simulink model "Remedy_WWTP"  (R2022a)
settings: Solver=ode23t  StartTime=0.0  StopTime=inf  FixedStep=1E-4  MaxStep=100  RelTol=1e-4  EnableMultiTasking=on
InitFcn:
  | iniASU_UNIT
undefined symbols (not defined in the file or in its folder): Arrhenius, Cineticos20, Esteq, Inf_Const, Param_ASU_D, Param_ASU_N, Param_Settler_Fns, ParamsEsteq, VarManip_D, VarManip_N, VarManip_QRF, x0_D, x0_N
libraries: modbusMatLib x3
settings Model: Creator=iirizar
settings SolverCC: InitialStep=1E-22  MaxConsecutiveMinStep=auto  AlgebraicLoopSolver=TrustRegion  SolverResetMethod=Robust
settings DataIOCC: LimitDataPoints=on  MaxDataPoints=1  SaveFinalState=on  SaveFormat=Array  SignalLoggingSaveFormat=ModelDataLogs  SaveOutput=off  SaveState=on  SignalLogging=off  SaveTime=off  ReturnWorkspaceOutputs=off
settings OptimizationCC: ExpressionDepthLimit=2147483647  LifeSpan=inf
settings DebuggingCC: UnderspecifiedInitializationDetection=Classic  MergeDetectMultiDrivingBlocksExec=none  SolverPrmCheckMsg=warning  FcnCallInpInsideContextMsg=warning  UnconnectedInputMsg=warning  UnconnectedOutputMsg=warning  UnconnectedLineMsg=warning  StateNameClashWarn=warning  SFUnexpectedBacktrackingDiag=warning  SFNoUnconditionalDefaultTransitionDiag=warning  SFExecutionAtInitializationDiag=none  SFMachineParentedDataDiag=warning  ArithmeticOperatorsInVariantConditions=warning
settings HardwareCC: ProdBitPerPointer=32  ProdBitPerSizeT=32  ProdBitPerPtrDiffT=32  ProdLargestAtomicFloat=None  ProdIntDivRoundTo=Undefined  ProdEndianess=Unspecified  ProdWordSize=32  ProdHWDeviceType=32-bit Generic
settings ModelReferenceCC: PropagateSignalLabelsOutOfModel=off
settings SFSimCC: SimUseLocalCustomCode=off  CustomCodeUndefinedFunction=UseInterfaceOnly
settings RTWCC: RTWUseLocalCustomCode=off  DLArmComputeVersion=19.05
settings CodeAppCC: StateflowObjectComments=on
settings GRTTargetCC: TargetLangStandard=C89/C90 (ANSI)  CombineOutputUpdateFcns=off  GRTInterface=on
settings ConfigComp: CovMetricSettings=dw  CovSaveCumulativeToWorkspaceVar=on  CovSaveSingleToWorkspaceVar=on  CovExternalEMLEnable=off

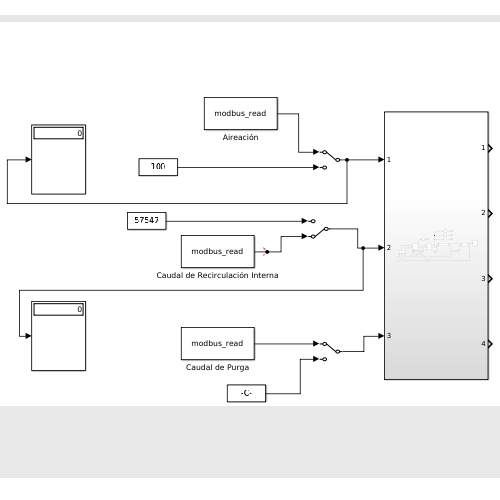
[thumbnail: Simulink's stored preview of the top-level diagram]
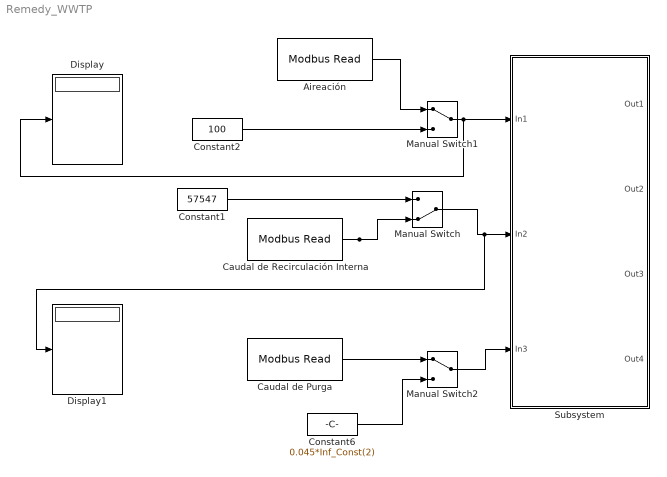
== system Remedy_WWTP ==
  Aireación : modbusMatLib/Modbus Read  registry=2065  ipAddress='openplc'  port=502
  Caudal de Purga : modbusMatLib/Modbus Read  registry=2069  ipAddress='openplc'  port=502
  Caudal de Recirculación Interna : modbusMatLib/Modbus Read  registry=2073  ipAddress='openplc'  port=502
  Constant1 : Constant  Value=57547
  Constant2 : Constant  Value=100
  Constant6 : Constant  Value=0.045*Inf_Const(2)
  Display : Display
  Display1 : Display
  Manual Switch : ManualSwitch  CurrentSetting=0
  Manual Switch1 : ManualSwitch
  Manual Switch2 : ManualSwitch
  Subsystem : Subsystem
  wires:
  Caudal de Recirculación Interna/1 -> Manual Switch/2
  Manual Switch/1 -> Display1/1, Subsystem/2(In2)
  Manual Switch1/1 -> Display/1, Subsystem/1(In1)
  Aireación/1 -> Manual Switch1/1
  Constant2/1 -> Manual Switch1/2
  Constant1/1 -> Manual Switch/1
  Caudal de Purga/1 -> Manual Switch2/1
  Constant6/1 -> Manual Switch2/2
  Manual Switch2/1 -> Subsystem/3(In3)

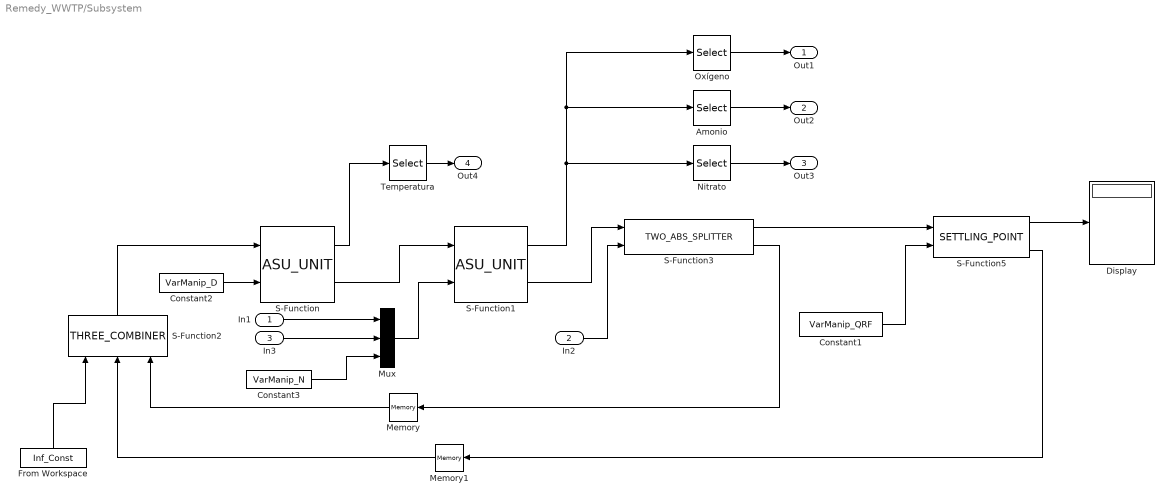
== system Remedy_WWTP/Subsystem ==
  In1 : Inport
  In2 : Inport  Port=2
  In3 : Inport  Port=3
  Amonio : Selector  InputPortWidth=9  IndexOptions=Index vector (dialog)  Indices=[4]  OutputSizes=1
  Constant1 : Constant  Value=VarManip_QRF
  Constant2 : Constant  Value=VarManip_D
  Constant3 : Constant  Value=VarManip_N
  Display : Display
  From Workspace : FromWorkspace  VariableName=Inf_Const  Interpolate=off  OutputAfterFinalValue=Holding final value
  Memory : Memory  InheritSampleTime=on
  Memory1 : Memory  InheritSampleTime=on
  Mux : Mux  Inputs=3
  Nitrato : Selector  InputPortWidth=9  IndexOptions=Index vector (dialog)  Indices=[3]  OutputSizes=1
  Oxígeno : Selector  InputPortWidth=9  IndexOptions=Index vector (dialog)  Indices=[5]  OutputSizes=1
  S-Function : S-Function  FunctionName=ASU_UNIT  Parameters=ParamsEsteq,Cineticos20,Arrhenius,Esteq,Param_ASU_D,x0_D  SFunctionDeploymentMode=off  EnableBusSupport=off
  S-Function1 : S-Function  FunctionName=ASU_UNIT  Parameters=ParamsEsteq,Cineticos20,Arrhenius,Esteq,Param_ASU_N,x0_N  SFunctionDeploymentMode=off  EnableBusSupport=off
  S-Function2 : S-Function  FunctionName=THREE_COMBINER  SFunctionDeploymentMode=off  EnableBusSupport=off
  S-Function3 : S-Function  FunctionName=TWO_ABS_SPLITTER  SFunctionDeploymentMode=off  EnableBusSupport=off
  S-Function5 : S-Function  FunctionName=SETTLING_POINT  Parameters=ParamsEsteq,Param_Settler_Fns  SFunctionDeploymentMode=off  EnableBusSupport=off
  Temperatura : Selector  InputPortWidth=9  IndexOptions=Index vector (dialog)  Indices=[8]  OutputSizes=1
  Out1 : Outport
  Out2 : Outport  Port=2
  Out3 : Outport  Port=3
  Out4 : Outport  Port=4
  wires:
  Constant2/1 -> S-Function/2
  Constant1/1 -> S-Function5/2
  In1/1 -> Mux/1
  Mux/1 -> S-Function1/2
  Constant3/1 -> Mux/3
  S-Function/2 -> S-Function1/1
  S-Function5/1 -> Display/1
  Memory1/1 -> S-Function2/2
  S-Function2/1 -> S-Function/1
  Memory/1 -> S-Function2/3
  S-Function5/3 -> Memory1/1
  S-Function1/2 -> S-Function3/1
  S-Function3/2 -> Memory/1
  S-Function3/1 -> S-Function5/1
  From Workspace/1 -> S-Function2/1
  In2/1 -> S-Function3/2
  In3/1 -> Mux/2
  S-Function1/1 -> Nitrato/1, Amonio/1, Oxígeno/1
  S-Function/1 -> Temperatura/1
  Nitrato/1 -> Out3/1
  Amonio/1 -> Out2/1
  Oxígeno/1 -> Out1/1
  Temperatura/1 -> Out4/1
